simulink model "videogradfilt"  (R2014b)
settings: Solver=ode45  StartTime=0.0  StopTime=10.0  RelTol=1e-3
libraries: dspvision x2
settings Model: Creator=Shogo  LastModifiedBy=Shogo

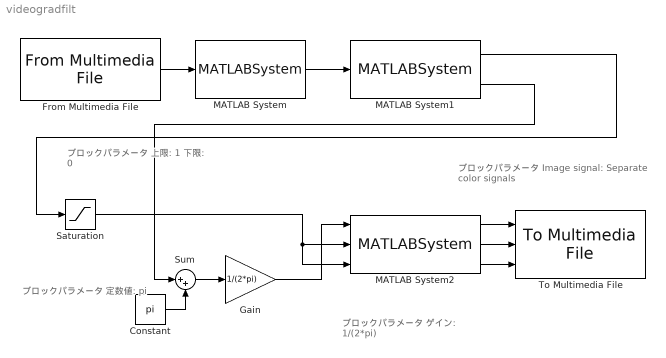
== system videogradfilt ==
  note: ブロックパラメータ
      | Image signal: Separate color signals
  note: ブロックパラメータ
      | 定数値: pi
  note: ブロックパラメータ
      | 上限: 1
      | 下限: 0
  note: ブロックパラメータ
      | ゲイン: 1/(2*pi)
  Constant : Constant  Value=pi
  From Multimedia File : dspvision/From Multimedia File  inputFilename=vipmen.avi  loop=on  numPlays=inf  outputStreams=Video only  videoDataType=single  audioDataType=int16  inheritSampleTime=on  userDefinedSampleTime=1/30  noAudioOutput=off  isIntensityVideo=off  fourcc=RGB  colorVideoFormat=One multidimensional signal  outputEOF=off  dataOrg=Column-major  audioFrameSize=1024  computeAudioFrameSize=off  outSamplingMode=Sample based
  Gain : Gain  Gain=1/(2*pi)
  MATLAB System : MATLABSystem  System=Rgb2GraySystem
      mask Type: Rgb2GraySystem
      mask Display:
      | disp('RGB to Gray');
      | port_label('input',1,'RGB');
      | port_label('output',1,'Gray');
  MATLAB System1 : MATLABSystem  System=GradFiltSystem  Kernel=[ 1, 1, 1; 0, 0, 0; -1, -1, -1 ]
      mask Type: GradFiltSystem
      mask Display:
      | disp('Grad. Filt.');
      | port_label('input',1,'Gray');
      | port_label('output',1,'Mag.');
      | port_label('output',2,'Ang.');
  MATLAB System2 : MATLABSystem  System=Hsv2RgbSystem
      mask Type: Hsv2RgbSystem
      mask Display:
      | disp('HSV to RGB');
      | port_label('input',1,'H');
      | port_label('input',2,'S');
      | port_label('input',3,'V');
      | port_label('output',1,'R');
      | port_label('output',2,'G');
      | port_label('output',3,'B');
  Saturation : Saturate  UpperLimit=1  LowerLimit=0
  Sum : Sum  Inputs=|++
  To Multimedia File : dspvision/To Multimedia File  outputFilename=vipmengradfilt.avi  streamSelection=Video only  videoCompressor=None (uncompressed)  audioCompressor=None (uncompressed)  imagePorts=Separate color signals  fileType=AVI  audioDatatype=Determine from input data type  fourcc=RGB  videoQuality=75  mj2000CompFactor=10
  wires:
  From Multimedia File/1 -> MATLAB System/1
  MATLAB System/1 -> MATLAB System1/1
  MATLAB System2/1 -> To Multimedia File/1
  MATLAB System2/2 -> To Multimedia File/2
  MATLAB System2/3 -> To Multimedia File/3
  MATLAB System1/1 -> Saturation/1
  Saturation/1 -> MATLAB System2/2, MATLAB System2/3
  Gain/1 -> MATLAB System2/1
  MATLAB System1/2 -> Sum/1
  Sum/1 -> Gain/1
  Constant/1 -> Sum/2
